simulink model "CASO_INSULINAS_DIFERENTES"  (R2019b)
settings: Solver=VariableStepAuto  StartTime=0.0  StopTime=50000  RelTol=1e-3
undefined symbols (not defined in the file): n, p1, p2, p3, p6, Vi
libraries: simulink x54
(part 1 of 2)
settings Model: Creator=USUARIO  LastModifiedBy=USUARIO

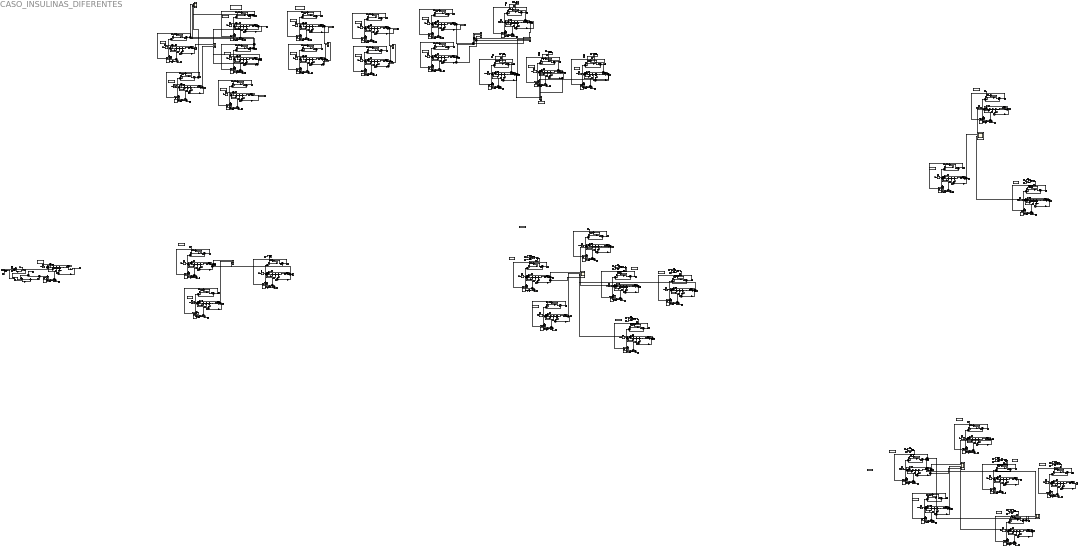
== system CASO_INSULINAS_DIFERENTES ==
  Clock{,1..43} (44 alike) : Clock
  Constant{1,3..4,6,9,11,13,15,17,19,21,23,25,27,29,31,33..34,37,39..40,42,44,46,50,55..56,58..59,61..62,64,66..67,71,74..75} (37 alike) : Constant  Value=0
  Constant{2,5,7..8,10,12,14,16,18,20,22,24,26,28,30,32,35..36,38,41,43,47,51,53..54,57,60,63,65,68,72,76,78} (33 alike) : Constant  Value=Vi
  Constant45 : Constant  Value=0.2
  Constant{48,52,69,73,77} (5 alike) : Constant  Value=0.1
  Constant49 : Constant  Value=0.2
  Constant70 : Constant  Value=0.2
  Divide{1..33} (33 alike) : Product  Inputs=*/
  GLUCOSA AYUNO1 : Scope  NumInputPorts=5
  Gain{1,5,8,10,14,19,24,27,32,34,39,41,46,48,50,54,59,62,64,68,73,76,78,83,85,90,92,97,99,103,108,110,115,117,122,124,129,131,136,138,143,145,150,152,157,159,164,166,171,173,178,180,185,187,192,194,199,201,206,208,213,215,220,222,227,229,231,236} (68 alike) : Gain  Gain=p1
  Gain{2,6,11,15,35,42,49,51,55,65,69,79,86,93,100,111,118,125,132,139,146,153,160,167,174,181,188,195,202,209,216,223,230,232} (34 alike) : Gain  Gain=p3
  Gain{3,7,12,16,18,21,23,26,29,31,36,38,43,45,52,56,58,61,66,70,72,75,80,82,87,89,94,96,101..102,105,107,112,114,119,121,126,128,133,135,140,142,147,149,154,156,161,163,168,170,175,177,182,184,189,191,196,198,203,205,210,212,217,219,224,226,233,235} (68 alike) : Gain  Gain=18
  Gain{9,20,25,28,33,40,47,60,63,74,77,84,91,98,104,109,116,123,130,137,144,151,158,165,172,179,186,193,200,207,214,221,228,237} (34 alike) : Gain  Gain=p2
  Gain{4,13,17,22,30,37,44,53,57,67,71,81,88,95,106,113,120,127,134,141,148,155,162,169,176,183,190,197,204,211,218,225,234} (33 alike) : Gain  Gain=n
  Glucosa 1 : Constant  Value=7
  Glucosa basal{1..13,16,21,24..42} (34 alike) : Constant  Value=7
  Glucosa basal14 : Constant  Value=0.25
  Glucosa basal{15,20,23,44} (4 alike) : Constant  Value=0
  Glucosa basal17 : Constant
  Glucosa basal18 : Constant  Value=0.25
  Glucosa basal19 : Constant  Value=0.25
  Glucosa basal22 : Constant
  Glucosa basal43 : Constant  Value=0.185
  Grafica ingesta D{1..34} (34 alike) : Scope
  INSULINA1 : Scope
  Ib1 : Constant  Value=10
  Ingesta 75 g1 : MATLAB Function  TreatAsAtomicUnit=on
  Ingesta 75 g10 : MATLAB Function  TreatAsAtomicUnit=on
  Ingesta 75 g11 : MATLAB Function  TreatAsAtomicUnit=on
  Ingesta 75 g12 : MATLAB Function  TreatAsAtomicUnit=on
  Ingesta 75 g13 : MATLAB Function  TreatAsAtomicUnit=on
  Ingesta 75 g14 : MATLAB Function  TreatAsAtomicUnit=on
  Ingesta 75 g15 : MATLAB Function  TreatAsAtomicUnit=on
  Ingesta 75 g16 : MATLAB Function  TreatAsAtomicUnit=on
  Ingesta 75 g17 : MATLAB Function  TreatAsAtomicUnit=on
  Ingesta 75 g18 : MATLAB Function  TreatAsAtomicUnit=on
  Ingesta 75 g19 : MATLAB Function  TreatAsAtomicUnit=on
  Ingesta 75 g2 : MATLAB Function  TreatAsAtomicUnit=on
  Ingesta 75 g20 : MATLAB Function  TreatAsAtomicUnit=on
  Ingesta 75 g21 : MATLAB Function  TreatAsAtomicUnit=on
  Ingesta 75 g22 : MATLAB Function  TreatAsAtomicUnit=on
  Ingesta 75 g23 : MATLAB Function  TreatAsAtomicUnit=on
  Ingesta 75 g24 : MATLAB Function  TreatAsAtomicUnit=on
  Ingesta 75 g25 : MATLAB Function  TreatAsAtomicUnit=on
  Ingesta 75 g26 : MATLAB Function  TreatAsAtomicUnit=on
  Ingesta 75 g27 : MATLAB Function  TreatAsAtomicUnit=on
  Ingesta 75 g28 : MATLAB Function  TreatAsAtomicUnit=on
  Ingesta 75 g29 : MATLAB Function  TreatAsAtomicUnit=on
  Ingesta 75 g3 : MATLAB Function  TreatAsAtomicUnit=on
  Ingesta 75 g30 : MATLAB Function  TreatAsAtomicUnit=on
  Ingesta 75 g31 : MATLAB Function  TreatAsAtomicUnit=on
  Ingesta 75 g32 : MATLAB Function  TreatAsAtomicUnit=on
  Ingesta 75 g33 : MATLAB Function  TreatAsAtomicUnit=on
  Ingesta 75 g34 : MATLAB Function  TreatAsAtomicUnit=on
  Ingesta 75 g4 : MATLAB Function  TreatAsAtomicUnit=on
  Ingesta 75 g5 : MATLAB Function  TreatAsAtomicUnit=on
  Ingesta 75 g6 : MATLAB Function  TreatAsAtomicUnit=on
  Ingesta 75 g7 : MATLAB Function  TreatAsAtomicUnit=on
  Ingesta 75 g8 : MATLAB Function  TreatAsAtomicUnit=on
  Ingesta 75 g9 : MATLAB Function  TreatAsAtomicUnit=on
  Insulina basal{1..34} (34 alike) : Constant  Value=10
  Integrator{1,4,7,10,13,16,22,25,28,31,34,55,58,61,64,67,70,76,79,85,91,94,97,100} (24 alike) : Integrator  InitialCondition=10
  Integrator{2,11,14,17,20,23,26,29,32,35,38,41,43,47,50,53,56,59,62,65,68,71,74,77,80,83,86,89,92,95,98,101} (32 alike) : Integrator  InitialCondition=7
  Integrator{3,6,9,12,15,18..19,24,27,30,36..37,40,44..46,49,52,57,60,63,69,72..73,78,81..82,87..88,93,96,99,102} (33 alike) : Integrator
  Integrator{21,33,39,42,48,51,54,66,75,84,90} (11 alike) : Integrator  InitialCondition=-0.000194
  Integrator5 : Integrator  InitialCondition=10.5
  Integrator8 : Integrator  InitialCondition=10.5
  Model Info1 : simulink/Model-Wide Utilities/Model Info  Frame=on  DisplayStringWithTags=|  HorizontalTextAlignment=Center  LeftAlignmentValue=0.5
      | MODELO MODIFICADO
      | 
      | AYUNAS CON INSULINA
      | 
      | PERSONA DIABETICA tipo 1
  Model Info10 : simulink/Model-Wide Utilities/Model Info  Frame=on  DisplayStringWithTags=|  HorizontalTextAlignment=Center  LeftAlignmentValue=0.5
      | MODELO MODIFICADO
      | 
      | INGESTA SIN INSULINA
      | 
      | PERSONA DIABETICA tipo 1
  Model Info11 : simulink/Model-Wide Utilities/Model Info  Frame=on  DisplayStringWithTags=|  HorizontalTextAlignment=Center  LeftAlignmentValue=0.5
      | MODELO MODIFICADO
      | 
      | TRAS INGESTA CON INSULINA
      | 
      | PERSONA DIABETICA
  Model Info12 : simulink/Model-Wide Utilities/Model Info  Frame=on  DisplayStringWithTags=|  HorizontalTextAlignment=Center  LeftAlignmentValue=0.5
      | MODELO MODIFICADO
      | 
      | INGESTA SIN INSULINA
      | 
      | PERSONA DIABETICA tipo 1
  Model Info13 : simulink/Model-Wide Utilities/Model Info  Frame=on  DisplayStringWithTags=|  HorizontalTextAlignment=Center  LeftAlignmentValue=0.5
      | MODELO MODIFICADO
      | 
      | TRAS INGESTA CON INSULINA
      | 
      | PERSONA DIABETICA
  Model Info14 : simulink/Model-Wide Utilities/Model Info  Frame=on  DisplayStringWithTags=|  HorizontalTextAlignment=Center  LeftAlignmentValue=0.5
      | INSULINA RAPIDA
      | 
      | CON DIFERENTES
      | TIPOS DE G DE INGESTA
  Model Info15 : simulink/Model-Wide Utilities/Model Info  Frame=on  DisplayStringWithTags=|  HorizontalTextAlignment=Center  LeftAlignmentValue=0.5
      | MODELO MODIFICADO
      | 
      | TRAS INGESTA CON INSULINA
      | 
      | PERSONA DIABETICA
  Model Info16 : simulink/Model-Wide Utilities/Model Info  Frame=on  DisplayStringWithTags=|  HorizontalTextAlignment=Center  LeftAlignmentValue=0.5
      | MODELO MODIFICADO
      | 
      | TRAS INGESTA CON INSULINA
      | 
      | PERSONA DIABETICA
  Model Info17 : simulink/Model-Wide Utilities/Model Info  Frame=on  DisplayStringWithTags=|  HorizontalTextAlignment=Center  LeftAlignmentValue=0.5
      | MODELO MODIFICADO
      | 
      | TRAS INGESTA CON INSULINA
      | 
      | PERSONA DIABETICA
  Model Info18 : simulink/Model-Wide Utilities/Model Info  Frame=on  DisplayStringWithTags=|  HorizontalTextAlignment=Center  LeftAlignmentValue=0.5
      | MODELO ORIGINAL
      | 
      | 
      | AYUNAS
      | 
      | PACIENTE DIABETICO
  Model Info19 : simulink/Model-Wide Utilities/Model Info  Frame=on  DisplayStringWithTags=INTENTO VARIAR LA INSULINA  HorizontalTextAlignment=Center  LeftAlignmentValue=0.5
  Model Info2 : simulink/Model-Wide Utilities/Model Info  Frame=on  DisplayStringWithTags=|  HorizontalTextAlignment=Center  LeftAlignmentValue=0.5
      | MODELO MODIFICADO
      | 
      | TRAS INGESTA SIN INSULINA
      | 
      | PERSONA DIABETICA tipo 1
  Model Info20 : simulink/Model-Wide Utilities/Model Info  Frame=on  DisplayStringWithTags=|  HorizontalTextAlignment=Center  LeftAlignmentValue=0.5
      | MODELO MODIFICADO
      | 
      | TRAS INGESTA CON INSULINA
      | 
      | PERSONA DIABETICA
  Model Info21 : simulink/Model-Wide Utilities/Model Info  Frame=on  DisplayStringWithTags=RAMPA 0.6 INSULINA + 0.1  HorizontalTextAlignment=Center  LeftAlignmentValue=0.5
  Model Info22 : simulink/Model-Wide Utilities/Model Info  Frame=on  DisplayStringWithTags=COMBINACION INSULINA RAPIDA Y PROLONGADA  HorizontalTextAlignment=Center  LeftAlignmentValue=0.5
  Model Info23 : simulink/Model-Wide Utilities/Model Info  Frame=on  DisplayStringWithTags=|  HorizontalTextAlignment=Center  LeftAlignmentValue=0.5
      | MODELO MODIFICADO
      | 
      | TRAS INGESTA CON INSULINA
      | 
      | PERSONA DIABETICA
  Model Info24 : simulink/Model-Wide Utilities/Model Info  Frame=on  DisplayStringWithTags=RAMPA 0.6  HorizontalTextAlignment=Center  LeftAlignmentValue=0.5
  Model Info25 : simulink/Model-Wide Utilities/Model Info  Frame=on  DisplayStringWithTags=RAMPA 0.3  HorizontalTextAlignment=Center  LeftAlignmentValue=0.5
  Model Info26 : simulink/Model-Wide Utilities/Model Info  Frame=on  DisplayStringWithTags=|  HorizontalTextAlignment=Center  LeftAlignmentValue=0.5
      | MODELO MODIFICADO
      | 
      | TRAS INGESTA CON INSULINA
      | 
      | PERSONA DIABETICA
  Model Info27 : simulink/Model-Wide Utilities/Model Info  Frame=on  DisplayStringWithTags=|  HorizontalTextAlignment=Center  LeftAlignmentValue=0.5
      | MODELO MODIFICADO
      | 
      | TRAS INGESTA CON INSULINA
      | 
      | PERSONA DIABETICA
  Model Info28 : simulink/Model-Wide Utilities/Model Info  Frame=on  DisplayStringWithTags=INTENTO VARIAR LA INSULINA  HorizontalTextAlignment=Center  LeftAlignmentValue=0.5
  Model Info29 : simulink/Model-Wide Utilities/Model Info  Frame=on  DisplayStringWithTags=RAMPA 0.6 INSULINA + 0.1  HorizontalTextAlignment=Center  LeftAlignmentValue=0.5
  Model Info3 : simulink/Model-Wide Utilities/Model Info  Frame=on  DisplayStringWithTags=|  HorizontalTextAlignment=Center  LeftAlignmentValue=0.5
      | MODELO MODIFICADO
      | 
      | TRAS INGESTA CON INSULINA
      | 
      | PERSONA DIABETICA
  Model Info30 : simulink/Model-Wide Utilities/Model Info  Frame=on  DisplayStringWithTags=INTENTO VARIAR LA INSULINA  HorizontalTextAlignment=Center  LeftAlignmentValue=0.5
  Model Info31 : simulink/Model-Wide Utilities/Model Info  Frame=on  DisplayStringWithTags=RAMPA 0.3  HorizontalTextAlignment=Center  LeftAlignmentValue=0.5
  Model Info32 : simulink/Model-Wide Utilities/Model Info  Frame=on  DisplayStringWithTags=|  HorizontalTextAlignment=Center  LeftAlignmentValue=0.5
      | MODELO MODIFICADO
      | 
      | TRAS INGESTA CON INSULINA
      | 
      | PERSONA DIABETICA
  Model Info33 : simulink/Model-Wide Utilities/Model Info  Frame=on  DisplayStringWithTags=RAMPA 0.6  HorizontalTextAlignment=Center  LeftAlignmentValue=0.5
  Model Info34 : simulink/Model-Wide Utilities/Model Info  Frame=on  DisplayStringWithTags=RAMPA 0.3  HorizontalTextAlignment=Center  LeftAlignmentValue=0.5
  Model Info35 : simulink/Model-Wide Utilities/Model Info  Frame=on  DisplayStringWithTags=|  HorizontalTextAlignment=Center  LeftAlignmentValue=0.5
      | CASO BUENO
      | 
      | INSULINAS RAPIDAS
  Model Info4 : simulink/Model-Wide Utilities/Model Info  Frame=on  DisplayStringWithTags=|  HorizontalTextAlignment=Center  LeftAlignmentValue=0.5
      | MODELO MODIFICADO
      | 
      | TRAS INGESTA CON INSULINA
      | 
      | PERSONA DIABETICA
  Model Info5 : simulink/Model-Wide Utilities/Model Info  Frame=on  DisplayStringWithTags=AYUNAS  HorizontalTextAlignment=Center  LeftAlignmentValue=0.5
  Model Info6 : simulink/Model-Wide Utilities/Model Info  Frame=on  DisplayStringWithTags=|  HorizontalTextAlignment=Center  LeftAlignmentValue=0.5
      | MODELO MODIFICADO
      | 
      | TRAS INGESTA CON INSULINA
      | 
      | PERSONA DIABETICA
  Model Info7 : simulink/Model-Wide Utilities/Model Info  Frame=on  DisplayStringWithTags=|  HorizontalTextAlignment=Center  LeftAlignmentValue=0.5
      | MODELO MODIFICADO
      | 
      | TRAS INGESTA CON INSULINA
      | 
      | PERSONA DIABETICA
  Model Info8 : simulink/Model-Wide Utilities/Model Info  Frame=on  DisplayStringWithTags=|  HorizontalTextAlignment=Center  LeftAlignmentValue=0.5
      | MODELO MODIFICADO
      | 
      | TRAS INGESTA CON INSULINA
      | 
      | PERSONA DIABETICA
  Model Info9 : simulink/Model-Wide Utilities/Model Info  Frame=on  DisplayStringWithTags=TRAS INGESTA  HorizontalTextAlignment=Center  LeftAlignmentValue=0.5
  Product{1..36} (36 alike) : Product
  Ramp : simulink/Sources/Ramp  slope=0.00033  start=10000  InitialOutput=0
  Rampa ascendente{,3..4,7..8} (5 alike) : simulink/Sources/Ramp  slope=0.000083  start=0  InitialOutput=0
  Rampa ascendente{1..2,5..6} (4 alike) : simulink/Sources/Ramp  slope=0.000166  start=0  InitialOutput=0
  Rampa descendente : simulink/Sources/Ramp  slope=-0.0000125  start=400*60  InitialOutput=0.3
  Rampa descendente1 : simulink/Sources/Ramp  slope=-0.000025  start=400*60  InitialOutput=0.6
  Rampa descendente2 : simulink/Sources/Ramp  slope=-0.000025  start=400*60  InitialOutput=0.6
  Rampa descendente3 : simulink/Sources/Ramp  slope=-0.0000125  start=400*60  InitialOutput=0.3
  Rampa descendente4 : simulink/Sources/Ramp  slope=-0.0000125  start=120*60  InitialOutput=0.3
  Rampa descendente5 : simulink/Sources/Ramp  slope=-0.000025  start=120*60  InitialOutput=0.6
  Rampa descendente6 : simulink/Sources/Ramp  slope=-0.000025  start=400*60  InitialOutput=0.6
  Rampa descendente7 : simulink/Sources/Ramp  slope=-0.0000125  start=500*60  InitialOutput=0.3
  Rampa descendente8 : simulink/Sources/Ramp  slope=-0.0000125  start=400*60  InitialOutput=0.3
  Saturation{,1,3,5,7,9,11,13,15,17} (10 alike) : Saturate  UpperLimit=0.3  LowerLimit=0
  Saturation{2,4,6,8,10,12,14,16,18} (9 alike) : Saturate  UpperLimit=0  LowerLimit=0
  Step{,1..2,5} (4 alike) : Step  Time=180*60  After=0.3  SampleTime=0
  Step3 : Step  Time=10  Before=7  After=4  SampleTime=0
  Step4 : Step  Time=10000  After=0.3  SampleTime=0
  Sum{1..2,4..6,8..11,13..15,17..29,31..35,37..41,43..44,46..48,50..56,58..60,62..68,70..74,76..80,82..85,87..97,99..103,105..108,110..114,116..119,121..126,128..132,134,136..139,141..142,144..146,148..152,154..157,159..164,166..170,172..176,178..184,186..188,190,192..195,197..202,204..205,207..209} (172 alike) : Sum  Inputs=|+-
  Sum{3,7,12,16,30,36,42,45,49,57,61,69,75,81,86,98,104,109,115,120,127,133,135,140,143,147,153,158,165,171,177,185,189,191,196,203,206} (37 alike) : Sum  Inputs=|++
  Switch{,5..7,10,12} (6 alike) : Switch  Criteria=u2 > Threshold  Threshold=400*60
  Switch1 : Switch  Criteria=u2 > Threshold  Threshold=6.67
  Switch11 : Switch  Criteria=u2 > Threshold  Threshold=500*60
  Switch13 : Switch  Criteria=u2 > Threshold  Threshold=6.67
  Switch2 : Switch  Criteria=u2 > Threshold  Threshold=11
  Switch3 : Switch  Criteria=u2 > Threshold  Threshold=5
  Switch4 : Switch  Criteria=u2 > Threshold  Threshold=6.67
  Switch8 : Switch  Criteria=u2 > Threshold  Threshold=120*60
  Switch9 : Switch  Criteria=u2 > Threshold  Threshold=120*60
  U (ins. exógena) cte{1..2,8,10} (4 alike) : Constant  Value=0
  U (ins. exógena) cte{3,7,9,11..14,19} (8 alike) : Constant  Value=0.185
  U (ins. exógena) cte15 : Constant  Value=0.3
  U (ins. exógena) cte{4,16..18} (4 alike) : Constant  Value=0.2
  U (ins. exógena) cte5 : Constant  Value=0.3
  U (ins. exógena) cte6 : Constant  Value=0.1
  glucoa en ayunas : Scope  NumInputPorts=2
  glucosa tras ingesta{1..13,15..33} (32 alike) : Scope  NumInputPorts=2
  glucosa tras ingesta14 : Scope  NumInputPorts=3
  grafica insulina{,1,3..4,6..10,12..17,19..20,22..24,26..31,33..34,36..40} (33 alike) : Scope  NumInputPorts=2
  grafica insulina11 : Scope  NumInputPorts=5
  grafica insulina18 : Scope  NumInputPorts=4
  grafica insulina2 : Scope  NumInputPorts=3
  grafica insulina21 : Scope  NumInputPorts=4
  grafica insulina25 : Scope  NumInputPorts=7
  grafica insulina32 : Scope  NumInputPorts=7
  grafica insulina35 : Scope  NumInputPorts=5
  grafica insulina41 : Scope  NumInputPorts=3
  grafica insulina42 : Scope  NumInputPorts=5
  grafica insulina5 : Scope  NumInputPorts=3
  insulina activa{1..34} (34 alike) : Scope
  mODELO ORIGINAL3 : Scope  NumInputPorts=2
  p1 : Constant  Value=5
  p2 : Gain  Gain=p6
  p4 = n1 : Gain  Gain=n
  wires:
  Gain12/1 -> glucosa tras ingesta2/1, grafica insulina2/1  "tras ingesta, paciente diabetico"
  Glucosa basal2/1 -> Gain8/1, Gain7/1  "glucosa basal"
  Sum19/1 -> Integrator7/1
  Product3/1 -> Sum8/2
  Sum15/1 -> Sum18/1
  U (ins. exógena) cte3/1 -> Divide3/1
  Gain9/1 -> Sum13/2
  Constant4/1 -> Grafica ingesta D2/1, Sum11/1
  Integrator9/1 -> insulina activa3/1, Product4/2, Gain20/1  "X(t)"
  Sum9/1 -> Integrator4/1
  Gain10/1 -> Sum11/2
  Gain8/1 -> Sum12/2
  Sum10/1 -> Gain11/1
  Sum14/1 -> Gain15/1
  U (ins. exógena) cte2/1 -> Divide2/1
  Gain7/1 -> glucosa tras ingesta2/2  "glucosa basal diabetico"
  Integrator6/1 -> insulina activa2/1, Product3/2, Gain9/1  "X(t)"
  Constant6/1 -> Grafica ingesta D3/1, Sum15/1
  Gain20/1 -> Sum17/2
  Sum8/1 -> Sum12/1
  Sum18/1 -> Sum16/1
  Divide3/1 -> Sum19/1
  Gain18/1 -> grafica insulina2/3, glucosa tras ingesta3/2  "glucosa basal"
  Clock2/1 -> Ingesta 75 g2/1(in)
  Insulina basal3/1 -> grafica insulina/2, Sum10/2  "insulina basal"
  Integrator8/1 -> Gain16/1, Product4/1, Gain14/1  "G(t)"
  Sum17/1 -> Integrator9/1
  Integrator5/1 -> Gain12/1, Product3/1, Gain10/1  "G(t)"
  Gain11/1 -> Sum13/1
  Sum16/1 -> Integrator8/1
  Glucosa basal3/1 -> Gain19/1, Gain18/1  "glucosa basal"
  Gain15/1 -> Sum17/1
  Gain16/1 -> grafica insulina2/2, glucosa tras ingesta3/1  "INGESTA CON INSULINA MOD"
  Gain19/1 -> Sum16/2
  Divide2/1 -> Sum9/1
  Integrator4/1 -> grafica insulina/1, Gain13/1, Sum10/1  "I(t)"
  Gain14/1 -> Sum15/2
  Sum11/1 -> Sum8/1
  Product4/1 -> Sum18/2
  Gain17/1 -> Sum19/2
  Insulina basal4/1 -> grafica insulina1/2, Sum14/2  "insulina basal"
  Gain13/1 -> Sum9/2
  Constant5/1 -> Divide2/2
  Constant7/1 -> Divide3/2
  Sum12/1 -> Integrator5/1
  Sum13/1 -> Integrator6/1
  Clock3/1 -> Ingesta 75 g3/1(in)
  Integrator7/1 -> grafica insulina1/1, Gain17/1, Sum14/1  "I(t)"
  Constant3/1 -> Grafica ingesta D4/1, Sum6/1
  Integrator3/1 -> insulina activa1/1, Product1/2, Gain28/1  "X(t)"
  Gain26/1 -> glucosa tras ingesta1/2  "glucosa basal diabetico"
  U (ins. exógena) cte1/1 -> Divide1/1
  Sum5/1 -> Gain6/1
  Gain27/1 -> Sum3/2
  Integrator12/1 -> insulina activa4/1, Product2/2, Gain25/1  "X(t)"
  Sum1/1 -> Gain2/1
  Sum24/1 -> Integrator1/1
  Gain1/1 -> Sum2/2
  Gain28/1 -> Sum4/2
  U (ins. exógena) cte4/1 -> Divide4/1
  Constant1/1 -> Grafica ingesta D1/1, Sum2/1
  Sum6/1 -> Sum21/1
  Product1/1 -> Sum23/2
  Gain3/1 -> GLUCOSA AYUNO1/1, glucosa tras ingesta1/1  "Glcuosa sin insulina exógena"
  Insulina basal1/1 -> grafica insulina3/2, Sum1/2  "insulina basal"
  Gain23/1 -> GLUCOSA AYUNO1/5, glucosa tras ingesta4/2  "glucosa basal"
  Sum20/1 -> Integrator12/1
  Sum22/1 -> Integrator10/1
  Divide4/1 -> Sum22/1
  Sum21/1 -> Sum7/1
  Clock1/1 -> Ingesta 75 g1/1(in)
  Gain25/1 -> Sum20/2
  Constant8/1 -> Divide4/2
  Sum3/1 -> Integrator2/1
  Integrator10/1 -> grafica insulina42/3, grafica insulina4/1, Gain22/1, Sum5/1  "Insulina con insulina exógena dosis media"
  Insulina basal2/1 -> grafica insulina4/2, grafica insulina42/5, Sum5/2  "insulina basal"
  Gain4/1 -> Sum24/2
  Sum4/1 -> Integrator3/1
  Product2/1 -> Sum21/2
  Gain22/1 -> Sum22/2
  Sum2/1 -> Sum23/1
  Sum23/1 -> Sum3/1
  Constant2/1 -> Divide1/2
  Gain5/1 -> Sum6/2
  Glucosa basal1/1 -> Gain27/1, Gain26/1  "glucosa basal"
  Integrator1/1 -> grafica insulina42/1, grafica insulina3/1, Gain4/1, Sum1/1  "Insulina sin insulina exógena"
  Integrator11/1 -> Gain21/1, Product2/1, Gain5/1  "G(t)"
  Gain24/1 -> Sum7/2
  Divide1/1 -> Sum24/1
  Gain21/1 -> GLUCOSA AYUNO1/3, glucosa tras ingesta4/1  "Glucosa con insulina exógena dosis media"
  Clock4/1 -> Ingesta 75 g4/1(in)
  Gain6/1 -> Sum20/1
  Sum7/1 -> Integrator11/1
  Gain2/1 -> Sum4/1
  Glucosa basal4/1 -> Gain24/1, Gain23/1  "glucosa basal"
  Integrator2/1 -> Gain3/1, Product1/1, Gain1/1  "G(t)"
  U (ins. exógena) cte5/1 -> Divide5/1
  Sum29/1 -> Sum26/1
  Glucosa basal5/1 -> Gain32/1, Gain31/1  "glucosa basal"
  Sum30/1 -> Integrator14/1
  Gain35/1 -> Sum25/1
  Clock5/1 -> Ingesta 75 g5/1(in)
  Gain29/1 -> GLUCOSA AYUNO1/4, glucosa tras ingesta5/1  "Glucosa con insulina exógena dosis alta"
  Gain32/1 -> Sum30/2
  Sum28/1 -> Gain35/1
  Integrator15/1 -> insulina activa5/1, Product5/2, Gain33/1  "X(t)"
  Integrator14/1 -> Gain29/1, Product5/1, Gain34/1  "G(t)"
  Constant10/1 -> Divide5/2
  Gain34/1 -> Sum29/2
  Gain30/1 -> Sum27/2
  Constant9/1 -> Grafica ingesta D5/1, Sum29/1
  Product5/1 -> Sum26/2
  Insulina basal5/1 -> grafica insulina6/2, Sum28/2  "insulina basal"
  Gain33/1 -> Sum25/2
  Integrator13/1 -> Gain30/1, Sum28/1, grafica insulina42/4, grafica insulina6/1  "Insulina con insulina exógena dosis alta"
  Gain31/1 -> glucosa tras ingesta5/2  "glucosa basal"
  Divide5/1 -> Sum27/1
  Sum27/1 -> Integrator13/1
  Sum25/1 -> Integrator15/1
  Sum26/1 -> Sum30/1
  U (ins. exógena) cte6/1 -> Divide6/1
  Sum35/1 -> Sum32/1
  Glucosa basal6/1 -> Gain39/1, Gain38/1  "glucosa basal"
  Sum36/1 -> Integrator17/1
  Gain42/1 -> Sum31/1
  Clock6/1 -> Ingesta 75 g6/1(in)
  Gain36/1 -> GLUCOSA AYUNO1/2, glucosa tras ingesta6/1  "Glucosa con insulina exógena dosis baja"
  Gain39/1 -> Sum36/2
  Sum34/1 -> Gain42/1
  Integrator18/1 -> insulina activa6/1, Product6/2, Gain40/1  "X(t)"
  Integrator17/1 -> Gain36/1, Product6/1, Gain41/1  "G(t)"
  Constant12/1 -> Divide6/2
  Gain41/1 -> Sum35/2
  Gain37/1 -> Sum33/2
  Constant11/1 -> Grafica ingesta D6/1, Sum35/1
  Product6/1 -> Sum32/2
  Insulina basal6/1 -> grafica insulina8/2, Sum34/2  "insulina basal"
  Gain40/1 -> Sum31/2
  Integrator16/1 -> grafica insulina42/2, grafica insulina8/1, Gain37/1, Sum34/1  "Insulina con insulina exógena dosis baja"
  Gain38/1 -> glucosa tras ingesta6/2  "glucosa basal"
  Divide6/1 -> Sum33/1
  Sum33/1 -> Integrator16/1
  Sum31/1 -> Integrator18/1
  Sum32/1 -> Sum36/1
  U (ins. exógena) cte7/1 -> Divide7/1
  Sum41/1 -> Sum38/1
  Glucosa basal7/1 -> Gain46/1, Gain45/1  "glucosa basal"
  Sum42/1 -> Integrator20/1
  Gain49/1 -> Sum37/1
  Clock7/1 -> Ingesta 75 g7/1(in)
  Gain43/1 -> glucoa en ayunas/1  "ayuno CON INSULINA insulina exacta"
  Gain46/1 -> Sum42/2
  Sum40/1 -> Gain49/1
  Integrator21/1 -> insulina activa7/1, Product7/2, Gain47/1  "X(t)"
  Integrator20/1 -> Gain43/1, Product7/1, Gain48/1  "G(t)"
  Constant14/1 -> Divide7/2
  Gain48/1 -> Sum41/2
  Gain44/1 -> Sum39/2
  Constant13/1 -> Grafica ingesta D7/1, Sum41/1
  Product7/1 -> Sum38/2
  Insulina basal7/1 -> grafica insulina7/2, Sum40/2  "insulina basal"
  Gain47/1 -> Sum37/2
  Integrator19/1 -> grafica insulina7/1, Gain44/1, Sum40/1  "I(t)"
  Gain45/1 -> glucoa en ayunas/2  "glucosa basal"
  Divide7/1 -> Sum39/1
  Sum39/1 -> Integrator19/1
  Sum37/1 -> Integrator21/1
  Sum38/1 -> Sum42/1
  Integrator24/1 -> insulina activa8/1, Product8/2, Gain63/1  "X(t)"
  Gain61/1 -> glucosa tras ingesta7/2  "glucosa basal diabetico"
  U (ins. exógena) cte8/1 -> Divide8/1
  Sum47/1 -> Gain55/1
  Gain62/1 -> Sum45/2
  Integrator27/1 -> insulina activa9/1, Product9/2, Gain60/1  "X(t)"
  Sum43/1 -> Gain51/1
  Sum54/1 -> Integrator22/1
  Gain50/1 -> Sum44/2
  Gain63/1 -> Sum46/2
  U (ins. exógena) cte9/1 -> Divide9/1
  Sum48/1 -> Sum51/1
  Product8/1 -> Sum53/2
  Gain52/1 -> grafica insulina5/1, glucosa tras ingesta7/1  "tras ingesta, paciente diabetico"
  Insulina basal8/1 -> grafica insulina9/2, Sum43/2  "insulina basal"
  Gain58/1 -> grafica insulina5/3, glucosa tras ingesta8/2  "glucosa basal"
  Sum50/1 -> Integrator27/1
  Sum52/1 -> Integrator25/1
  Divide9/1 -> Sum52/1
  Sum51/1 -> Sum49/1
  Clock8/1 -> Ingesta 75 g8/1(in)
  Gain60/1 -> Sum50/2
  Constant18/1 -> Divide9/2
  Sum45/1 -> Integrator23/1
  Integrator25/1 -> grafica insulina10/1, Gain57/1, Sum47/1  "I(t)"
  Insulina basal9/1 -> grafica insulina10/2, Sum47/2  "insulina basal"
  Gain53/1 -> Sum54/2
  Sum46/1 -> Integrator24/1
  Product9/1 -> Sum51/2
  Gain57/1 -> Sum52/2
  Sum44/1 -> Sum53/1
  Sum53/1 -> Sum45/1
  Constant16/1 -> Divide8/2
  Gain54/1 -> Sum48/2
  Glucosa basal8/1 -> Gain62/1, Gain61/1  "glucosa basal"
  Integrator22/1 -> grafica insulina9/1, Gain53/1, Sum43/1  "I(t)"
  Integrator26/1 -> Gain56/1, Product9/1, Gain54/1  "G(t)"
  Gain59/1 -> Sum49/2
  Divide8/1 -> Sum54/1
  Gain56/1 -> grafica insulina5/2, glucosa tras ingesta8/1  "INGESTA CON INSULINA MOD"
  Clock9/1 -> Ingesta 75 g9/1(in)
  Gain55/1 -> Sum50/1
  Sum49/1 -> Integrator26/1
  Gain51/1 -> Sum46/1
  Glucosa basal9/1 -> Gain59/1, Gain58/1  "glucosa basal"
  Integrator23/1 -> Gain52/1, Product8/1, Gain50/1  "G(t)"
  Ingesta 75 g8/1(D) -> Grafica ingesta D8/1, Sum44/1
  Ingesta 75 g9/1(D) -> Grafica ingesta D9/1, Sum48/1
  Gain76/1 -> Sum57/2
  Sum59/1 -> Gain69/1
  Gain75/1 -> glucosa tras ingesta9/2  "glucosa basal diabetico"
  Integrator30/1 -> insulina activa10/1, Product10/2, Gain77/1  "X(t)"
  Ingesta 75 g11/1(D) -> Grafica ingesta D11/1, Sum60/1
  Ingesta 75 g10/1(D) -> Grafica ingesta D10/1, Sum56/1
  Integrator28/1 -> grafica insulina14/1, Gain67/1, Sum55/1  "I(t)"
  Glucosa basal10/1 -> Gain76/1, Gain75/1  "glucosa basal"
  U (ins. exógena) cte10/1 -> Divide10/1
  Gain68/1 -> Sum60/2
  Sum65/1 -> Sum57/1
  Constant20/1 -> Divide10/2
  Sum56/1 -> Sum65/1
  Product11/1 -> Sum63/2
  Insulina basal11/1 -> grafica insulina12/2, Sum59/2  "insulina basal"
  Sum58/1 -> Integrator30/1
  Gain71/1 -> Sum64/2
  Gain67/1 -> Sum66/2
  Integrator31/1 -> grafica insulina12/1, Gain71/1, Sum59/1  "I(t)"
  Sum57/1 -> Integrator29/1
  Gain72/1 -> glucosa tras ingesta14/3, grafica insulina11/5, glucosa tras ingesta10/2  "glucosa basal"
  Insulina basal10/1 -> grafica insulina14/2, Sum55/2  "insulina basal"
  Gain66/1 -> glucosa tras ingesta9/1, grafica insulina11/1, glucosa tras ingesta14/1  "INGESTA PACIENTE DIABETICO"
  Gain77/1 -> Sum58/2
  Gain64/1 -> Sum56/2
  Sum66/1 -> Integrator28/1
  Sum55/1 -> Gain65/1
  U (ins. exógena) cte11/1 -> Divide11/1
  Integrator33/1 -> insulina activa11/1, Product11/2, Gain74/1  "X(t)"
  Glucosa basal11/1 -> Gain73/1, Gain72/1  "glucosa basal"
  Clock10/1 -> Ingesta 75 g10/1(in)
  Sum63/1 -> Sum61/1
  Gain70/1 -> grafica insulina11/2, glucosa tras ingesta14/2, glucosa tras ingesta10/1  "INGESTA CON INSULINA"
  Divide11/1 -> Sum64/1
  Sum61/1 -> Integrator32/1
  Gain69/1 -> Sum62/1
  Clock11/1 -> Ingesta 75 g11/1(in)
  Sum64/1 -> Integrator31/1
  Gain65/1 -> Sum58/1
  Product10/1 -> Sum65/2
  Sum62/1 -> Integrator33/1
  Gain74/1 -> Sum62/2
  Integrator32/1 -> Gain70/1, Product11/1, Gain68/1  "G(t)"
  Gain73/1 -> Sum61/2
  Divide10/1 -> Sum66/1
  Sum60/1 -> Sum63/1
  Constant22/1 -> Divide11/2
  Integrator29/1 -> Gain66/1, Product10/1, Gain64/1  "G(t)"
  Gain83/1 -> Sum69/2
  Gain84/1 -> Sum70/2
  Constant24/1 -> Divide12/2
  Sum68/1 -> Sum71/1
  Glucosa basal12/1 -> Gain83/1, Gain82/1  "glucosa basal"
  Integrator36/1 -> insulina activa12/1, Product12/2, Gain84/1  "X(t)"
  Switch4/1 -> Divide12/1
  Sum71/1 -> Sum69/1
  Gain82/1 -> glucosa tras ingesta11/2  "glucosa basal"
  Integrator34/1 -> grafica insulina15/1, Gain81/1, Sum67/1  "I(t)"
  Gain81/1 -> Sum72/2
  Insulina basal12/1 -> grafica insulina15/2, Sum67/2  "insulina basal"
  Product12/1 -> Sum71/2
  Gain78/1 -> Sum68/2
  Ingesta 75 g12/1(D) -> Grafica ingesta D12/1, Sum68/1
  Sum67/1 -> Gain79/1
  Sum70/1 -> Integrator36/1
  Divide12/1 -> Sum72/1
  Sum69/1 -> Integrator35/1
  Gain79/1 -> Sum70/1
  Gain80/1 -> grafica insulina18/1, grafica insulina11/3, glucosa tras ingesta11/1  "INGESTA 50 g CON INSULINA RÁPIDA"
  Sum72/1 -> Integrator34/1
  Clock12/1 -> Ingesta 75 g12/1(in)
  Glucosa basal19/1 -> Switch4/1  "glucosa basal"
  Glucosa basal20/1 -> Switch4/3  "glucosa basal"
  Integrator35/1 -> Gain80/1, Switch4/2, Product12/1, Gain78/1  "G(t)"
  Sum74/1 -> Sum77/1
  Glucosa basal13/1 -> Gain90/1, Gain89/1  "glucosa basal"
  Gain91/1 -> Sum76/2
  Gain90/1 -> Sum75/2
  Integrator38/1 -> Gain87/1, Switch1/2, Product13/1, Gain85/1  "G(t)"
  Sum73/1 -> Gain86/1
  Gain85/1 -> Sum74/2
  Insulina basal13/1 -> grafica insulina16/2, Sum73/2  "insulina basal"
  Product13/1 -> Sum77/2
  Gain88/1 -> Sum78/2
  Integrator37/1 -> grafica insulina16/1, Gain88/1, Sum73/1  "I(t)"
  Gain89/1 -> grafica insulina18/4, glucosa tras ingesta12/2  "glucosa basal"
  Sum77/1 -> Sum75/1
  Ingesta 75 g13/1(D) -> Grafica ingesta D13/1, Sum74/1
  Integrator39/1 -> insulina activa13/1, Product13/2, Gain91/1  "X(t)"
  Gain87/1 -> grafica insulina18/2, glucosa tras ingesta12/1  "INGESTA 75 g CON INSULINA RÁPIDA"
  Clock13/1 -> Ingesta 75 g13/1(in)
  Sum78/1 -> Integrator37/1
  Divide13/1 -> Sum78/1
  Sum76/1 -> Integrator39/1
  Glucosa basal14/1 -> Switch1/1  "glucosa basal"
  Constant26/1 -> Divide13/2
  Sum75/1 -> Integrator38/1
  Gain86/1 -> Sum76/1
  Glucosa basal15/1 -> Switch1/3  "glucosa basal"
  Switch1/1 -> Divide13/1
  Sum80/1 -> Sum83/1
  Glucosa basal16/1 -> Gain97/1, Gain96/1  "glucosa basal"
  Gain98/1 -> Sum82/2
  Gain97/1 -> Sum81/2
  Integrator41/1 -> Gain94/1, Switch2/2, Product14/1, Gain92/1  "G(t)"
  Sum79/1 -> Gain93/1
  Gain92/1 -> Sum80/2
  Insulina basal14/1 -> grafica insulina17/2, Sum79/2  "insulina basal"
  Product14/1 -> Sum83/2
  Gain95/1 -> Sum84/2
  Integrator40/1 -> grafica insulina17/1, Gain95/1, Sum79/1  "I(t)"
  Gain96/1 -> glucosa tras ingesta13/2  "glucosa basal"
  Sum83/1 -> Sum81/1
  Ingesta 75 g14/1(D) -> Grafica ingesta D14/1, Sum80/1
  Integrator42/1 -> insulina activa14/1, Product14/2, Gain98/1  "X(t)"
  Gain94/1 -> grafica insulina18/3, glucosa tras ingesta13/1  "INGESTA 100 g CON INSULINA RÁPIDA"
  Clock14/1 -> Ingesta 75 g14/1(in)
  Sum84/1 -> Integrator40/1
  Divide14/1 -> Sum84/1
  Sum82/1 -> Integrator42/1
  Glucosa basal17/1 -> Switch2/1  "glucosa basal"
  Constant28/1 -> Divide14/2
  Sum81/1 -> Integrator41/1
  Gain93/1 -> Sum82/1
  Glucosa basal18/1 -> Switch2/3  "glucosa basal"
  Switch2/1 -> Divide14/1
  Sum92/1 -> Gain100/1
  Insulina basal15/1 -> Sum92/2  "insulina basal"
  Switch3/1 -> Product17/2
  Glucosa basal23/1 -> Switch3/3  "glucosa basal"
  Product16/1 -> Product17/1
  Gain99/1 -> Sum85/2
  Clock16/1 -> Ingesta 75 g15/1(in)
  Gain100/1 -> Sum90/1
  Glucosa basal22/1 -> Switch3/1  "glucosa basal"
  Integrator43/1 -> Gain101/1, Sum87/1, Switch3/2, Product15/1, Gain99/1  "G(t)"
  Gain103/1 -> Sum86/2
  Clock15/1 -> Product16/1
  Ib1/1 -> Sum88/2  "glucosa basal"
  Integrator45/1 -> insulina activa15/1, Product15/2, Gain104/1  "X(t)"
  Sum85/1 -> Sum91/1
  Product15/1 -> Sum91/2
  Product17/1 -> Sum89/1
  p1/1 -> Sum87/2  "glucosa basal"
  Gain102/1 -> mODELO ORIGINAL3/2  "glucosa basal"
  Sum88/1 -> p4 = n1/1
  p4 = n1/1 -> Sum89/2
  p2/1 -> Product16/2
  Sum91/1 -> Sum86/1
  Sum90/1 -> Integrator45/1
  Constant29/1 -> Grafica ingesta D15/1, Sum85/1
  Glucosa basal21/1 -> Gain103/1, Gain102/1  "glucosa basal"
  Sum86/1 -> Integrator43/1
  Gain104/1 -> Sum90/2
  Sum87/1 -> p2/1
  Integrator44/1 -> INSULINA1/1, Sum88/1, Sum92/1  "I(t)"
  Gain101/1 -> mODELO ORIGINAL3/1  "Glucosa tras ingesta con insulina modelada"
  Sum89/1 -> Integrator44/1
  Clock17/1 -> Ingesta 75 g16/1(in)
  Sum95/1 -> Integrator46/1
  Sum93/1 -> Integrator48/1
  Constant30/1 -> Divide15/2
  Gain108/1 -> Sum98/2
  Integrator51/1 -> insulina activa17/1, Product19/2, Gain116/1  "X(t)"
  Gain114/1 -> grafica insulina21/4, glucosa tras ingesta16/2  "glucosa basal"
  Gain116/1 -> Sum99/2
  Gain105/1 -> grafica insulina21/2, glucosa tras ingesta15/1  "AYUNO CON INSULINA 0.3 mg"
  Sum101/1 -> Integrator49/1
  Divide15/1 -> Sum95/1
  Gain110/1 -> Sum97/2
  Gain115/1 -> Sum104/2
  Sum94/1 -> Sum98/1
  Glucosa basal25/1 -> Gain115/1, Gain114/1  "glucosa basal"
  Integrator48/1 -> insulina activa16/1, Product18/2, Gain109/1  "X(t)"
  Integrator50/1 -> Gain112/1, Product19/1, Gain117/1  "G(t)"
  Sum103/1 -> Sum100/1
  Sum99/1 -> Integrator51/1
  Insulina basal17/1 -> grafica insulina20/2, Sum102/2  "insulina basal"
  Gain109/1 -> Sum93/2
  Product19/1 -> Sum100/2
  Sum102/1 -> Gain118/1
  Constant32/1 -> Divide16/2
  Gain113/1 -> Sum101/2
  Gain112/1 -> grafica insulina21/1, glucosa tras ingesta16/1  "AYUNO CON INSULINA ESCALON"
  Gain117/1 -> Sum103/2
  Sum98/1 -> Integrator47/1
  Integrator47/1 -> Gain105/1, Product18/1, Gain110/1  "G(t)"
  Gain107/1 -> glucosa tras ingesta15/2  "glucosa basal"
  Clock18/1 -> Ingesta 75 g17/1(in)
  Insulina basal16/1 -> grafica insulina19/2, Sum96/2  "insulina basal"
  Product18/1 -> Sum94/2
  Ingesta 75 g16/1(D) -> Grafica ingesta D16/1, Sum97/1
  Sum96/1 -> Gain111/1
  Ingesta 75 g17/1(D) -> Grafica ingesta D17/1, Sum103/1
  Gain111/1 -> Sum93/1
  Gain118/1 -> Sum99/1
  Gain106/1 -> Sum95/2
  Step4/1 -> Divide16/1
  U (ins. exógena) cte15/1 -> Divide15/1
  Sum104/1 -> Integrator50/1
  Glucosa basal24/1 -> Gain108/1, Gain107/1  "glucosa basal"
  Sum97/1 -> Sum94/1
  Integrator46/1 -> grafica insulina19/1, Gain106/1, Sum96/1  "I(t)"
  Integrator49/1 -> grafica insulina20/1, Gain113/1, Sum102/1  "I(t)"
  Sum100/1 -> Sum104/1
  Divide16/1 -> Sum101/1
  Ramp/1 -> Saturation/1
  Ingesta 75 g18/1(D) -> Grafica ingesta D18/1, Sum108/1
  Gain125/1 -> Sum110/1
  Gain122/1 -> Sum109/2
  Sum106/1 -> Integrator52/1
  Gain123/1 -> Sum110/2
  Gain121/1 -> glucosa tras ingesta17/2  "glucosa basal"
  Integrator54/1 -> insulina activa18/1, Product20/2, Gain123/1  "X(t)"
  Sum105/1 -> Sum109/1
  Divide17/1 -> Sum106/1
  Clock19/1 -> Ingesta 75 g18/1(in)
  Glucosa basal26/1 -> Gain122/1, Gain121/1  "glucosa basal"
  Gain124/1 -> Sum108/2
  Gain119/1 -> grafica insulina21/3, glucosa tras ingesta17/1  "AYUNO CON INSULINA RAMPA"
  Gain120/1 -> Sum106/2
  Sum107/1 -> Gain125/1
  Constant35/1 -> Divide17/2
  Sum109/1 -> Integrator53/1
  Product20/1 -> Sum105/2
  Insulina basal18/1 -> grafica insulina22/2, Sum107/2  "insulina basal"
  Sum108/1 -> Sum105/1
  Integrator53/1 -> Gain119/1, Product20/1, Gain124/1  "G(t)"
  Sum110/1 -> Integrator54/1
  Integrator52/1 -> grafica insulina22/1, Gain120/1, Sum107/1  "I(t)"
  Saturation/1 -> Divide17/1
  Switch/1 -> Sum135/1  "entrada U"
  Integrator61/1 -> grafica insulina26/1, Gain141/1, Sum118/1  "I(t)"
  Clock22/1 -> Ingesta 75 g21/1(in)
  Sum126/1 -> Sum123/1
  Sum121/1 -> Integrator63/1
  Integrator62/1 -> Gain140/1, Product23/1, Gain145/1  "G(t)"
  Gain141/1 -> Sum117/2
  Gain127/1 -> Sum124/2
  Sum119/1 -> Sum116/1
  Gain145/1 -> Sum119/2
  Gain143/1 -> Sum120/2
  U (ins. exógena) cte16/1 -> Divide18/1
  Integrator57/1 -> insulina activa19/1, Product21/2, Gain130/1  "X(t)"
  Product23/1 -> Sum116/2
  Sum125/1 -> Gain132/1
  Insulina basal21/1 -> grafica insulina26/2, Sum118/2  "insulina basal"
  Sum118/1 -> Gain146/1
  Gain140/1 -> grafica insulina25/6, glucosa tras ingesta20/1  "RAMPA 0.3 + 0.2"
  Gain131/1 -> Sum126/2
  Sum120/1 -> Integrator62/1
  Sum122/1 -> Integrator57/1
  Glucosa basal29/1 -> Gain143/1, Gain142/1  "glucosa basal"
  Constant41/1 -> Divide20/2
  Ingesta 75 g21/1(D) -> Grafica ingesta D21/1, Sum119/1
  Rampa ascendente/1 -> Saturation1/1
  Sum116/1 -> Sum120/1
  Integrator63/1 -> insulina activa21/1, Product23/2, Gain144/1  "X(t)"
  Divide20/1 -> Sum117/1
  Gain144/1 -> Sum121/2
  Gain146/1 -> Sum121/1
  Sum117/1 -> Integrator61/1
  Ingesta 75 g19/1(D) -> Grafica ingesta D19/1, Sum126/1
  Gain132/1 -> Sum122/1
  Clock20/1 -> Ingesta 75 g19/1(in)
  Gain142/1 -> glucosa tras ingesta20/2  "glucosa basal"
  Gain126/1 -> grafica insulina25/3, glucosa tras ingesta18/1  "INSULINA 0.2"
  Sum123/1 -> Sum127/1
  Integrator56/1 -> Gain126/1, Product21/1, Gain131/1  "G(t)"
  Integrator55/1 -> grafica insulina23/1, Gain127/1, Sum125/1  "I(t)"
  Gain128/1 -> glucosa tras ingesta18/2  "glucosa basal"
  Sum127/1 -> Integrator56/1
  Glucosa basal27/1 -> Gain129/1, Gain128/1  "glucosa basal"
  Gain130/1 -> Sum122/2
  Divide18/1 -> Sum124/1
  Constant36/1 -> Divide18/2
  Insulina basal19/1 -> grafica insulina23/2, Sum125/2  "insulina basal"
  Sum124/1 -> Integrator55/1
  Product21/1 -> Sum123/2
  Gain129/1 -> Sum127/2
  Rampa descendente/1 -> Saturation2/1
  Saturation2/1 -> Switch/1
  Saturation1/1 -> Switch/3
  Clock/1 -> Switch/2
  Sum130/1 -> Integrator64/1
  Gain153/1 -> Sum134/1
  Integrator64/1 -> grafica insulina27/1, Gain148/1, Sum131/1  "I(t)"
  Sum129/1 -> Sum133/1
  Integrator65/1 -> Gain147/1, Product24/1, Gain152/1  "G(t)"
  Insulina basal22/1 -> grafica insulina27/2, Sum131/2  "insulina basal"
  Gain152/1 -> Sum132/2
  Gain149/1 -> glucosa tras ingesta21/2  "glucosa basal"
  Constant44/1 -> Divide21/1
  Constant43/1 -> Divide21/2
  Sum133/1 -> Integrator65/1
  Product24/1 -> Sum129/2
  Sum132/1 -> Sum129/1
  Sum134/1 -> Integrator66/1
  Ingesta 75 g22/1(D) -> Grafica ingesta D22/1, Sum132/1
  Gain150/1 -> Sum133/2
  Glucosa basal30/1 -> Gain150/1, Gain149/1  "glucosa basal"
  Integrator66/1 -> insulina activa22/1, Product24/2, Gain151/1  "X(t)"
  Divide21/1 -> Sum130/1
  Gain151/1 -> Sum134/2
  Sum131/1 -> Gain153/1
  Gain148/1 -> Sum130/2
  Gain147/1 -> grafica insulina25/1, glucosa tras ingesta21/1  "INGESTA SIN INSULINA"
  Clock23/1 -> Ingesta 75 g22/1(in)
  Constant45/1 -> Sum135/2
  Sum135/1 -> Divide20/1
  Saturation3/1 -> Switch5/3
  Clock24/1 -> Switch5/2
  Saturation4/1 -> Switch5/1
  Rampa descendente1/1 -> Saturation4/1
  Constant47/1 -> Divide22/2
  Sum138/1 -> Gain160/1
  Sum140/1 -> Integrator68/1
  Gain156/1 -> glucosa tras ingesta22/2  "glucosa basal"
  Gain160/1 -> Sum141/1
  Divide22/1 -> Sum137/1
  Integrator69/1 -> insulina activa23/1, Product25/2, Gain158/1  "X(t)"
  Rampa ascendente1/1 -> Saturation3/1
  Sum136/1 -> Sum140/1
  Gain155/1 -> Sum137/2
  Integrator68/1 -> Gain154/1, Product25/1, Gain159/1  "G(t)"
  Sum137/1 -> Integrator67/1
  Sum139/1 -> Sum136/1
  Sum141/1 -> Integrator69/1
  Switch5/1 -> Divide22/1  "entrada U"
  Clock25/1 -> Ingesta 75 g23/1(in)
  Integrator67/1 -> grafica insulina28/1, Gain155/1, Sum138/1  "I(t)"
  Glucosa basal31/1 -> Gain157/1, Gain156/1  "glucosa basal"
  Product25/1 -> Sum136/2
  Gain157/1 -> Sum140/2
  Gain158/1 -> Sum141/2
  Insulina basal23/1 -> grafica insulina28/2, Sum138/2  "insulina basal"
  Gain159/1 -> Sum139/2
  Ingesta 75 g23/1(D) -> Grafica ingesta D23/1, Sum139/1
  Gain154/1 -> grafica insulina25/4, glucosa tras ingesta22/1  "RAMPA 0.6"
  Saturation5/1 -> Switch6/3
  Clock21/1 -> Switch6/2
  Saturation6/1 -> Switch6/1
  Rampa descendente2/1 -> Saturation6/1
  Constant38/1 -> Divide19/2
  Sum113/1 -> Gain139/1
  Sum115/1 -> Integrator59/1
  Gain135/1 -> grafica insulina25/7, glucosa tras ingesta19/2  "glucosa basal"
  Gain139/1 -> Sum128/1
  Divide19/1 -> Sum112/1
  Integrator60/1 -> insulina activa20/1, Product22/2, Gain137/1  "X(t)"
  Rampa ascendente2/1 -> Saturation5/1
  Sum111/1 -> Sum115/1
  Constant49/1 -> Sum143/2
  Gain134/1 -> Sum112/2
  Integrator59/1 -> Gain133/1, Product22/1, Gain138/1  "G(t)"
  Sum112/1 -> Integrator58/1
  Sum114/1 -> Sum111/1
  Sum128/1 -> Integrator60/1
  Switch6/1 -> Sum143/1  "entrada U"
  Clock26/1 -> Ingesta 75 g20/1(in)
  Integrator58/1 -> grafica insulina24/1, Gain134/1, Sum113/1  "I(t)"
  Glucosa basal28/1 -> Gain136/1, Gain135/1  "glucosa basal"
  Product22/1 -> Sum111/2
  Gain136/1 -> Sum115/2
  Gain137/1 -> Sum128/2
  Insulina basal20/1 -> grafica insulina24/2, Sum113/2  "insulina basal"
  Gain138/1 -> Sum114/2
  Ingesta 75 g20/1(D) -> Grafica ingesta D20/1, Sum114/1
  Gain133/1 -> grafica insulina25/2, glucosa tras ingesta19/1  "RAMPA 0.6 +0.2"
  Sum143/1 -> Divide19/1
  Gain167/1 -> Sum148/1
  Divide23/1 -> Sum144/1
  Sum145/1 -> Gain167/1
  Sum147/1 -> Integrator71/1
  Saturation8/1 -> Switch7/1
  Rampa descendente3/1 -> Saturation8/1
  Constant51/1 -> Divide23/2
  Saturation7/1 -> Switch7/3
  Clock27/1 -> Switch7/2
  Gain163/1 -> glucosa tras ingesta23/2  "glucosa basal"
  Insulina basal24/1 -> grafica insulina29/2, Sum145/2  "insulina basal"
  Gain165/1 -> Sum148/2
  Product26/1 -> Sum142/2
  Gain166/1 -> Sum146/2
  Glucosa basal32/1 -> Gain164/1, Gain163/1  "glucosa basal"
  Ingesta 75 g24/1(D) -> Grafica ingesta D24/1, Sum146/1
  Gain164/1 -> Sum147/2
  Sum144/1 -> Integrator70/1
  Integrator71/1 -> Gain161/1, Product26/1, Gain166/1  "G(t)"
  Integrator70/1 -> grafica insulina29/1, Gain162/1, Sum145/1  "I(t)"
  Gain161/1 -> grafica insulina25/5, glucosa tras ingesta23/1  "RAMPA 0.3"
  Sum148/1 -> Integrator72/1
  Clock28/1 -> Ingesta 75 g24/1(in)
  Integrator72/1 -> insulina activa24/1, Product26/2, Gain165/1  "X(t)"
  Switch7/1 -> Divide23/1  "entrada U"
  Gain162/1 -> Sum144/2
  Sum146/1 -> Sum142/1
  Sum142/1 -> Sum147/1
  Rampa ascendente3/1 -> Saturation7/1
  Sum167/1 -> Sum171/1
  Integrator82/1 -> grafica insulina34/1, Gain190/1, Sum169/1  "I(t)"
  Constant61/1 -> Divide27/1
  Gain189/1 -> grafica insulina32/1, glucosa tras ingesta27/1  "INGESTA SIN INSULINA"
  Clock33/1 -> Ingesta 75 g28/1(in)
  Gain190/1 -> Sum168/2
  Sum169/1 -> Gain195/1
  Divide27/1 -> Sum168/1
  Gain193/1 -> Sum172/2
  Integrator84/1 -> insulina activa28/1, Product30/2, Gain193/1  "X(t)"
  Rampa ascendente7/1 -> Saturation15/1
  Sum180/1 -> Sum185/1
  Gain204/1 -> Sum182/2
  Sum184/1 -> Sum180/1
  Switch11/1 -> Divide29/1  "entrada U"
  Gain203/1 -> grafica insulina32/5, glucosa tras ingesta29/1  "RAMPA 0.3"
  Sum186/1 -> Integrator90/1
  Clock38/1 -> Ingesta 75 g30/1(in)
  Integrator89/1 -> Gain203/1, Product32/1, Gain208/1  "G(t)"
  Gain207/1 -> Sum186/2
  Gain208/1 -> Sum184/2
  Glucosa basal38/1 -> Gain206/1, Gain205/1  "glucosa basal"
  Product32/1 -> Sum180/2
  Constant68/1 -> Divide29/2
  Rampa descendente7/1 -> Saturation16/1
  Insulina basal30/1 -> grafica insulina36/2, Sum183/2  "insulina basal"
  Gain205/1 -> glucosa tras ingesta29/2  "glucosa basal"
  Saturation15/1 -> Switch11/3
  Sum185/1 -> Integrator89/1
  Sum183/1 -> Gain209/1
  Saturation16/1 -> Switch11/1
  Gain209/1 -> Sum186/1
  Gain195/1 -> Sum172/1
  Sum168/1 -> Integrator82/1
  Gain173/1 -> Sum164/2
  Divide29/1 -> Sum182/1
  Sum160/1 -> Integrator75/1
  Gain174/1 -> Sum160/1
  Clock30/1 -> Ingesta 75 g25/1(in)
  Integrator90/1 -> insulina activa30/1, Product32/2, Gain207/1  "X(t)"
  Gain206/1 -> Sum185/2
  Integrator88/1 -> grafica insulina36/1, Gain204/1, Sum183/1  "I(t)"
  Divide24/1 -> Sum162/1
  Gain172/1 -> Sum160/2
  Sum165/1 -> Integrator74/1
  Integrator73/1 -> grafica insulina30/1, Gain169/1, Sum163/1  "I(t)"
  Glucosa basal33/1 -> Gain171/1, Gain170/1  "glucosa basal"
  Gain170/1 -> glucosa tras ingesta24/2  "glucosa basal"
  Sum161/1 -> Sum165/1
  Product27/1 -> Sum161/2
  Constant53/1 -> Divide24/2
  Gain169/1 -> Sum162/2
  Sum162/1 -> Integrator73/1
  Integrator74/1 -> Gain168/1, Product27/1, Gain173/1  "G(t)"
  Sum163/1 -> Gain174/1
  Sum182/1 -> Integrator88/1
  Integrator75/1 -> insulina activa25/1, Product27/2, Gain172/1  "X(t)"
  U (ins. exógena) cte17/1 -> Divide24/1
  Product30/1 -> Sum167/2
  Constant60/1 -> Divide27/2
  Gain194/1 -> Sum170/2
  Glucosa basal36/1 -> Gain192/1, Gain191/1  "glucosa basal"
  Sum164/1 -> Sum161/1
  Gain192/1 -> Sum171/2
  Ingesta 75 g28/1(D) -> Grafica ingesta D28/1, Sum170/1
  Sum172/1 -> Integrator84/1
  Ingesta 75 g30/1(D) -> Grafica ingesta D30/1, Sum184/1
  Sum170/1 -> Sum167/1
  Insulina basal25/1 -> grafica insulina30/2, Sum163/2  "insulina basal"
  Gain191/1 -> glucosa tras ingesta27/2  "glucosa basal"
  Gain171/1 -> Sum165/2
  Integrator83/1 -> Gain189/1, Product30/1, Gain194/1  "G(t)"
  Gain168/1 -> grafica insulina32/3, glucosa tras ingesta24/1  "INSULINA 0.2"
  Ingesta 75 g25/1(D) -> Grafica ingesta D25/1, Sum164/1
  Sum171/1 -> Integrator83/1
  Insulina basal28/1 -> grafica insulina34/2, Sum169/2  "insulina basal"
  Clock37/1 -> Switch11/2
  Sum179/1 -> Sum189/1
  Integrator91/1 -> grafica insulina38/1, Gain211/1, Sum187/1  "I(t)"
  Saturation9/1 -> Switch8/3
  Constant70/1 -> Sum191/2
  Gain223/1 -> Sum197/1
  Sum194/1 -> Gain223/1
  Sum196/1 -> Integrator95/1
  Constant72/1 -> Divide31/2
  Clock36/1 -> Switch9/2
  Constant66/1 -> Divide30/1
  Integrator79/1 -> grafica insulina41/1, grafica insulina33/1, Gain183/1, Sum151/1  "Insulina exógena (dosis alta)"
  Switch10/1 -> Divide26/1  "entrada U"
  Clock40/1 -> Ingesta 75 g27/1(in)
  Sum152/1 -> Sum149/1
  Sum178/1 -> Integrator81/1
  Sum150/1 -> Integrator79/1
  Integrator80/1 -> Gain182/1, Product29/1, Gain187/1  "G(t)"
  Rampa descendente5/1 -> Saturation12/1
  Sum149/1 -> Sum153/1
  Sum153/1 -> Integrator80/1
  Gain188/1 -> Sum178/1
  Clock32/1 -> Switch10/2
  Saturation13/1 -> Switch10/3
  Sum151/1 -> Gain188/1
  Constant57/1 -> Divide26/2
  Saturation14/1 -> Switch10/1
  Rampa descendente6/1 -> Saturation14/1
  Gain182/1 -> grafica insulina35/2, glucosa tras ingesta26/1  "RAMPA 0.6"
  Ingesta 75 g27/1(D) -> Grafica ingesta D27/1, Sum152/1
  Product29/1 -> Sum149/2
  Glucosa basal35/1 -> Gain185/1, Gain184/1  "glucosa basal"
  Switch8/1 -> Sum191/1  "entrada U"
  Insulina basal32/1 -> grafica insulina39/2, Sum194/2  "insulina basal"
  Gain221/1 -> Sum197/2
  Product34/1 -> Sum192/2
  Gain220/1 -> Sum196/2
  Ingesta 75 g32/1(D) -> Grafica ingesta D32/1, Sum195/1
  Sum193/1 -> Integrator94/1
  Sum197/1 -> Integrator96/1
  Clock39/1 -> Ingesta 75 g32/1(in)
  Sum195/1 -> Sum192/1
  Gain218/1 -> Sum193/2
  Integrator96/1 -> insulina activa32/1, Product34/2, Gain221/1  "X(t)"
  Sum192/1 -> Sum196/1
  Integrator81/1 -> insulina activa27/1, Product29/2, Gain186/1  "X(t)"
  Gain210/1 -> grafica insulina35/1, glucosa tras ingesta30/1  "INGESTA SIN INSULINA"
  Clock35/1 -> Ingesta 75 g31/1(in)
  Integrator95/1 -> Gain217/1, Product34/1, Gain222/1  "G(t)"
  Integrator94/1 -> grafica insulina39/1, Gain218/1, Sum194/1  "I(t)"
  Gain211/1 -> Sum181/2
  Sum187/1 -> Gain216/1
  Divide30/1 -> Sum181/1
  Gain214/1 -> Sum190/2
  Integrator93/1 -> insulina activa31/1, Product33/2, Gain214/1  "X(t)"
  Rampa ascendente8/1 -> Saturation17/1
  Sum198/1 -> Sum203/1
  Gain225/1 -> Sum200/2
  Sum202/1 -> Sum198/1
  Switch12/1 -> Divide32/1  "entrada U"
  Saturation12/1 -> Switch9/1
  Gain224/1 -> grafica insulina35/4, glucosa tras ingesta32/1  "RAMPA 0.3"
  Sum204/1 -> Integrator99/1
  Clock42/1 -> Ingesta 75 g33/1(in)
  Integrator98/1 -> Gain224/1, Product35/1, Gain229/1  "G(t)"
  Gain187/1 -> Sum152/2
  Gain228/1 -> Sum204/2
  Gain229/1 -> Sum202/2
  Glucosa basal41/1 -> Gain227/1, Gain226/1  "glucosa basal"
  Product35/1 -> Sum198/2
  Constant76/1 -> Divide32/2
  Rampa descendente8/1 -> Saturation18/1
  Insulina basal33/1 -> grafica insulina40/2, Sum201/2  "insulina basal"
  Gain226/1 -> glucosa tras ingesta32/2  "glucosa basal"
  Saturation11/1 -> Switch9/3
  Saturation17/1 -> Switch12/3
  Glucosa basal40/1 -> Gain220/1, Gain219/1  "glucosa basal"
  Sum203/1 -> Integrator98/1
  Sum201/1 -> Gain230/1
  Saturation18/1 -> Switch12/1
  Insulina basal27/1 -> grafica insulina41/3, grafica insulina33/2, Sum151/2  "insulina basal"
  Gain230/1 -> Sum204/1
  Saturation10/1 -> Switch8/1
  Rampa descendente4/1 -> Saturation10/1
  Gain216/1 -> Sum190/1
  Sum181/1 -> Integrator91/1
  Constant63/1 -> Divide28/2
  Glucosa basal37/1 -> Gain199/1, Gain198/1  "glucosa basal"
  Gain180/1 -> Sum176/2
  Sum156/1 -> Gain202/1
  Divide32/1 -> Sum200/1
  Sum166/1 -> Integrator78/1
  Sum158/1 -> Integrator86/1
  Gain196/1 -> glucosa tras ingesta28/1  "RAMPA 0.3 + 0.2"
  Gain181/1 -> Sum166/1
  Clock31/1 -> Ingesta 75 g26/1(in)
  Sum155/1 -> Integrator85/1
  Gain198/1 -> glucosa tras ingesta28/2  "glucosa basal"
  Integrator99/1 -> insulina activa33/1, Product35/2, Gain228/1  "X(t)"
  Gain200/1 -> Sum159/2
  Divide28/1 -> Sum155/1
  Integrator87/1 -> insulina activa29/1, Product31/2, Gain200/1  "X(t)"
  Gain227/1 -> Sum203/2
  Divide26/1 -> Sum150/1
  Rampa ascendente4/1 -> Saturation9/1
  Integrator97/1 -> grafica insulina41/2, grafica insulina40/1, Gain225/1, Sum201/1  "Insulina exógena (dosis baja)"
  Ingesta 75 g29/1(D) -> Grafica ingesta D29/1, Sum157/1
  Sum154/1 -> Sum158/1
  Gain222/1 -> Sum195/2
  Divide25/1 -> Sum174/1
  Gain179/1 -> Sum166/2
  Gain219/1 -> glucosa tras ingesta31/2  "glucosa basal"
  Sum177/1 -> Integrator77/1
  Integrator76/1 -> grafica insulina31/1, Gain176/1, Sum175/1  "I(t)"
  Glucosa basal34/1 -> Gain178/1, Gain177/1  "glucosa basal"
  Gain177/1 -> glucosa tras ingesta25/2  "glucosa basal"
  Sum173/1 -> Sum177/1
  Product28/1 -> Sum173/2
  Constant54/1 -> Divide25/2
  Gain197/1 -> Sum155/2
  Integrator86/1 -> Gain196/1, Product31/1, Gain201/1  "G(t)"
  Sum157/1 -> Sum154/1
  Gain176/1 -> Sum174/2
  Sum174/1 -> Integrator76/1
  Integrator77/1 -> Gain175/1, Product28/1, Gain180/1  "G(t)"
  Sum159/1 -> Integrator87/1
  Clock34/1 -> Ingesta 75 g29/1(in)
  Integrator85/1 -> grafica insulina37/1, Gain197/1, Sum156/1  "I(t)"
  Divide31/1 -> Sum193/1
  Insulina basal29/1 -> grafica insulina37/2, Sum156/2  "insulina basal"
  Sum175/1 -> Gain181/1
  Product31/1 -> Sum154/2
  Sum200/1 -> Integrator97/1
  Gain183/1 -> Sum150/2
  Integrator78/1 -> insulina activa26/1, Product28/2, Gain179/1  "X(t)"
  Gain217/1 -> glucosa tras ingesta31/1  "RAMPA 0.6"
  Gain199/1 -> Sum158/2
  Gain201/1 -> Sum157/2
  U (ins. exógena) cte18/1 -> Divide25/1
  Clock29/1 -> Switch8/2
  Product33/1 -> Sum179/2
  Constant65/1 -> Divide30/2
  Gain215/1 -> Sum188/2
  Glucosa basal39/1 -> Gain213/1, Gain212/1  "glucosa basal"
  Gain186/1 -> Sum178/2
  Rampa ascendente6/1 -> Saturation13/1
  Sum176/1 -> Sum173/1
  Gain213/1 -> Sum189/2
  Ingesta 75 g31/1(D) -> Grafica ingesta D31/1, Sum188/1
  Sum190/1 -> Integrator93/1
  Gain185/1 -> Sum153/2
  Ingesta 75 g33/1(D) -> Grafica ingesta D33/1, Sum202/1
  Sum188/1 -> Sum179/1
  Switch9/1 -> Divide31/1  "entrada U"
  Insulina basal26/1 -> grafica insulina31/2, Sum175/2  "insulina basal"
  Gain212/1 -> glucosa tras ingesta30/2  "glucosa basal"
  Gain202/1 -> Sum159/1
  Gain178/1 -> Sum177/2
  Integrator92/1 -> Gain210/1, Product33/1, Gain215/1  "G(t)"
  Rampa ascendente5/1 -> Saturation11/1
  Sum191/1 -> Divide28/1
  Gain184/1 -> grafica insulina35/5, glucosa tras ingesta26/2  "glucosa basal"
  Gain175/1 -> grafica insulina35/3, glucosa tras ingesta25/1  "INSULINA 0.2"
  Ingesta 75 g26/1(D) -> Grafica ingesta D26/1, Sum176/1
  Sum189/1 -> Integrator92/1
  Insulina basal31/1 -> grafica insulina38/2, Sum187/2  "insulina basal"
  Clock41/1 -> Switch12/2
  Sum205/1 -> Sum208/1
  Product36/1 -> Sum208/2
  Integrator101/1 -> Gain233/1, Switch13/2, Product36/1, Gain231/1  "G(t)"
  Insulina basal34/1 -> grafica insulina13/2, Sum199/2  "insulina basal"
  Sum199/1 -> Gain232/1
  Gain233/1 -> grafica insulina11/4, glucosa tras ingesta33/1  "Ingesta con insulina rápida (misma dosis)"
  Clock43/1 -> Ingesta 75 g34/1(in)
  Gain234/1 -> Sum209/2
  Sum209/1 -> Integrator100/1
  Integrator100/1 -> grafica insulina13/1, Gain234/1, Sum199/1  "I(t)"
  Gain232/1 -> Sum207/1
  Gain235/1 -> glucosa tras ingesta33/2  "glucosa basal"
  Gain237/1 -> Sum207/2
  Switch13/1 -> Divide33/1
  Divide33/1 -> Sum209/1
  Glucosa basal42/1 -> Gain236/1, Gain235/1  "glucosa basal"
  Sum208/1 -> Sum206/1
  Gain236/1 -> Sum206/2
  Glucosa basal43/1 -> Switch13/1  "glucosa basal"
  Integrator102/1 -> insulina activa34/1, Product36/2, Gain237/1  "X(t)"
  Ingesta 75 g34/1(D) -> Grafica ingesta D34/1, Sum205/1
  Sum207/1 -> Integrator102/1
  Constant78/1 -> Divide33/2
  Gain231/1 -> Sum205/2
  Glucosa basal44/1 -> Switch13/3  "glucosa basal"
  Sum206/1 -> Integrator101/1
